simulink model "arc"  (R2025b)
settings: Solver=VariableStepAuto  StartTime=0.0  StopTime=0.1  RelTol=1e-3
model mask{K1=K1, K2=K2, lambda=lambda, Xd=Xd, rd=rd, f=f, U_PhaseRMS=U_PhaseRMS}
model workspace (MAT data in the model file):
  K1 = 221320
  K2 = 0.00072
  U_PhaseRMS = 243
  Xd = 0.003
  f = 50
  lambda = 2
  rd = 0.0004
settings Model: ParameterArgumentNames=K1,K2,U_PhaseRMS,Xd,f,lambda,rd  Creator=LYG  LastModifiedBy=LYG

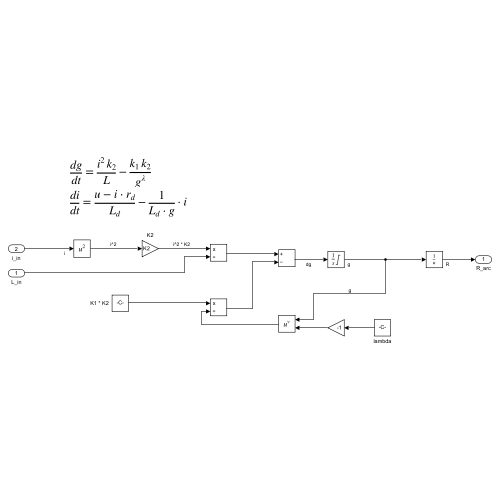
[thumbnail: Simulink's stored preview of the top-level diagram]
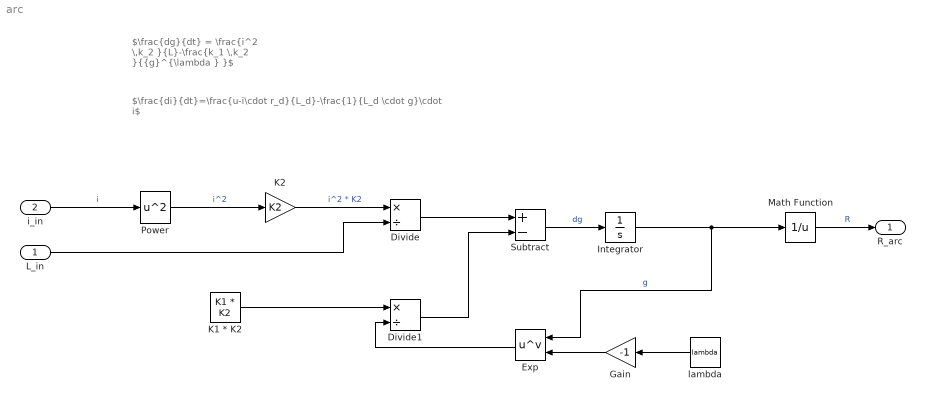
== system arc ==
  note: $\frac{di}{dt}=\frac{u-i\cdot r_d}{L_d}-\frac{1}{L_d \cdot g}\cdot i$
  note: $\frac{dg}{dt} = \frac{i^2 \,k_2 }{L}-\frac{k_1 \,k_2 }{{g}^{\lambda } }$
  L_in : Inport
  i_in : Inport  Port=2
  Divide : Product  Inputs=*/
  Divide1 : Product  Inputs=*/
  Exp : Math  Operator=pow
  Gain : Gain  Gain=-1
  Integrator : Integrator  InitialCondition=50  LimitOutput=on  UpperSaturationLimit=1e3  LowerSaturationLimit=1e-3
  K1 * K2 : Constant  Value=K1 * K2
  K2 : Gain  Gain=K2
  Math Function : Math  Operator=reciprocal
  Power : Math  Operator=square
  Subtract : Sum  Inputs=+-
  lambda : Constant  Value=lambda
  R_arc : Outport
  wires:
  Subtract/1 -> Integrator/1  "dg"
  Power/1 -> K2/1  "i^2"
  K2/1 -> Divide/1  "i^2 * K2"
  Divide/1 -> Subtract/1
  K1 * K2/1 -> Divide1/1
  Divide1/1 -> Subtract/2
  Integrator/1 -> Math Function/1, Exp/1  "g"
  Exp/1 -> Divide1/2
  lambda/1 -> Gain/1
  i_in/1 -> Power/1  "i"
  Math Function/1 -> R_arc/1  "R"
  Gain/1 -> Exp/2
  L_in/1 -> Divide/2
